simulink model "hybrid_ems"  (R2026a)
settings: Solver=ode45  StopTime=604800  FixedStep=3600

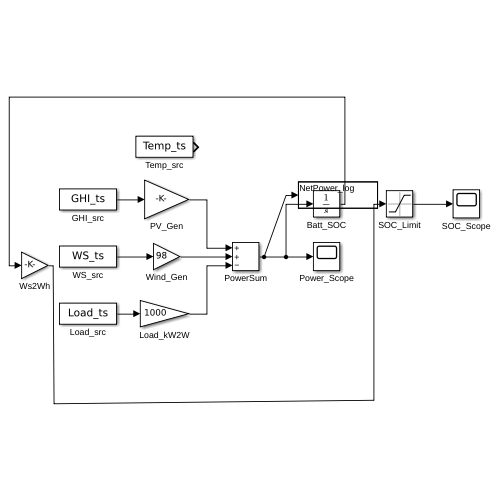
[thumbnail: Simulink's stored preview of the top-level diagram]
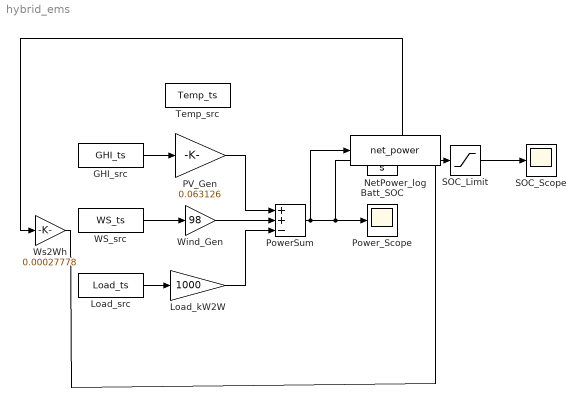
== system hybrid_ems ==
  Batt_SOC : Integrator  InitialCondition=25000*3600
  GHI_src : FromWorkspace  VariableName=GHI_ts
  Load_kW2W : Gain  Gain=1000
  Load_src : FromWorkspace  VariableName=Load_ts
  NetPower_log : ToWorkspace  VariableName=net_power  SampleTime=-1
  PV_Gen : Gain  Gain=0.063126
  PowerSum : Sum  Inputs=++-
  Power_Scope : Scope
      settings: ActiveDisplayYMinimum=-3145.5805223583075  ActiveDisplayYMaximum=3305.179037956279
  SOC_Limit : Saturate  UpperLimit=50000  LowerLimit=10000
  SOC_Scope : Scope
      settings: ActiveDisplayYMinimum=3357.6249855180686  ActiveDisplayYMaximum=28727.917447890988
  Temp_src : FromWorkspace  VariableName=Temp_ts
  WS_src : FromWorkspace  VariableName=WS_ts
  Wind_Gen : Gain  Gain=98
  Ws2Wh : Gain  Gain=0.00027778
  wires:
  Load_kW2W/1 -> PowerSum/3
  PV_Gen/1 -> PowerSum/1
  Load_src/1 -> Load_kW2W/1
  WS_src/1 -> Wind_Gen/1
  PowerSum/1 -> Power_Scope/1, Batt_SOC/1, NetPower_log/1
  Wind_Gen/1 -> PowerSum/2
  GHI_src/1 -> PV_Gen/1
  Batt_SOC/1 -> Ws2Wh/1
  Ws2Wh/1 -> SOC_Limit/1
  SOC_Limit/1 -> SOC_Scope/1
